simulink model "full car model"  (R2026a)
settings: Solver=VariableStepAuto  StopTime=10
settings Model: Creator=ANDALIBM  LastModifiedBy=eonra
settings SimscapeCC: SimscapeNominalValues="[{\"value\":\"1\",\"unit\":\"A\"},{\"value\":\"1\",\"unit\":\"bar\"},{\"value\":\"1\",\"unit\":\"cm^2\"},{\"value\":\"1\",\"unit\":\"cm^3/s\"},{\"value\":\"1\",\"unit\":\"kJ/kg\"},{\"value\":\"1\",\"unit\":\"kW\"},{\"value\":\"1\",\"unit\":\"l\"},{\"value\":\"1\",\"unit\":\"N\"},{\"value\":\"1\",\"unit\":\"N*m\"},{\"value\":\"1\",\"unit\":\"V\"}]"  SimscapeLogType=none  SimscapeLogDecimation=1  SimscapeLogDataHistory=5000

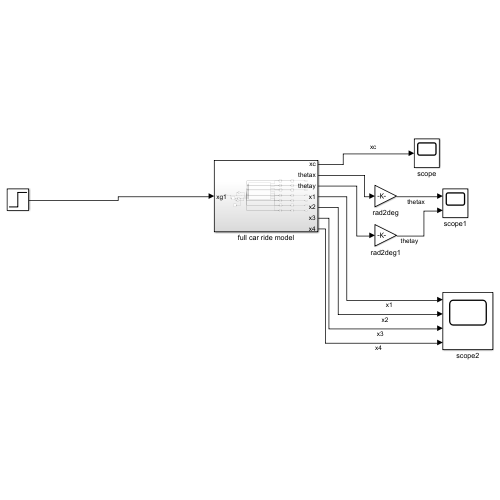
[thumbnail: Simulink's stored preview of the top-level diagram]
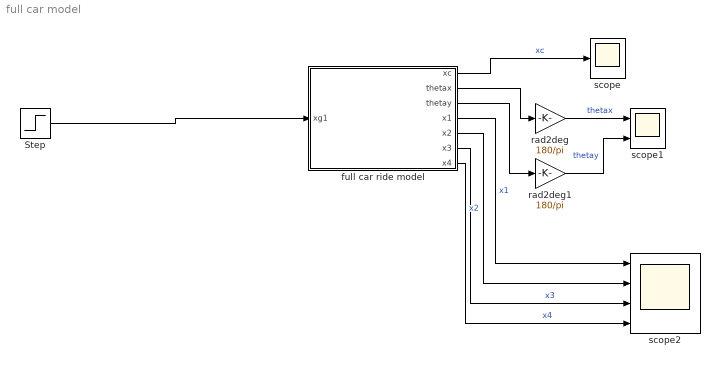
== system full car model ==
  Step : Step  FinalValue=0.05  SampleTime=0
  full car ride model : Subsystem
  rad2deg : Gain  Gain=180/pi
  rad2deg1 : Gain  Gain=180/pi
  scope : Scope
      settings: SampleTime=0.01  ActiveDisplayYMinimum=-0.0065929622757647608  ActiveDisplayYMaximum=0.01986979326753685  DataLoggingVariableName=xc  DataLoggingSaveFormat=Array
  scope1 : Scope  NumInputPorts=2
      settings: SampleTime=0.01  ActiveDisplayYMinimum=-2.6712831731592193  ActiveDisplayYMaximum=0.29680924146213544  DataLoggingSaveFormat=Structure
  scope2 : Scope  NumInputPorts=4
      settings: SampleTime=0.01  ActiveDisplayYMinimum=-0.025734237976273319  ActiveDisplayYMaximum=0.08318787384082596  DataLoggingVariableName=ScopeData2  DataLoggingSaveFormat=Structure
  wires:
  full car ride model/1(xc) -> scope/1  "xc"
  full car ride model/2(thetax) -> rad2deg/1
  rad2deg/1 -> scope1/1  "thetax"
  full car ride model/3(thetay) -> rad2deg1/1
  rad2deg1/1 -> scope1/2  "thetay"
  full car ride model/4(x1) -> scope2/1  "x1"
  full car ride model/7(x4) -> scope2/4  "x4"
  full car ride model/6(x3) -> scope2/3  "x3"
  full car ride model/5(x2) -> scope2/2  "x2"
  Step/1 -> full car ride model/1(xg1)

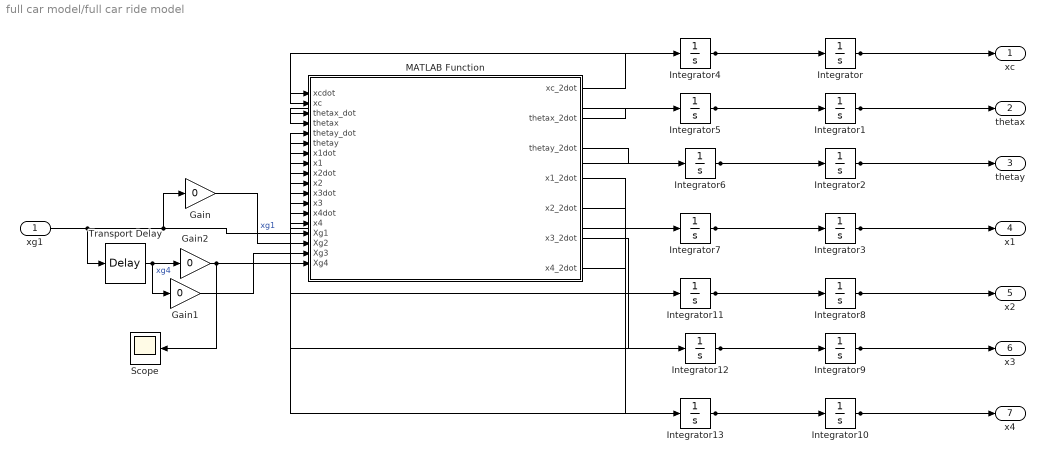
== system full car model/full car ride model ==
  xg1 : Inport
  Gain : Gain  Gain=0
  Gain1 : Gain  Gain=0
  Gain2 : Gain  Gain=0
  Integrator{,1..13} (14 alike) : Integrator
  MATLAB Function : MATLAB Function  TreatAsAtomicUnit=on
  Scope : Scope
      settings: ActiveDisplayYMinimum=-0.0089  ActiveDisplayYMaximum=0.28771  DataLoggingVariableName=ScopeData3
  Transport Delay : TransportDelay  DelayTime=3.1/5
  xc : Outport
  thetax : Outport  Port=2
  thetay : Outport  Port=3
  x1 : Outport  Port=4
  x2 : Outport  Port=5
  x3 : Outport  Port=6
  x4 : Outport  Port=7
  wires:
  Integrator/1 -> xc/1, MATLAB Function/2(xc)
  Integrator1/1 -> thetax/1, MATLAB Function/4(thetax)
  Integrator2/1 -> thetay/1, MATLAB Function/6(thetay)
  Integrator3/1 -> x1/1, MATLAB Function/8(x1)
  Integrator7/1 -> Integrator3/1, MATLAB Function/7(x1dot)
  Integrator6/1 -> Integrator2/1, MATLAB Function/5(thetay_dot)
  Integrator5/1 -> Integrator1/1, MATLAB Function/3(thetax_dot)
  Integrator4/1 -> Integrator/1, MATLAB Function/1(xcdot)
  xg1/1 -> Gain/1, MATLAB Function/15(Xg1), Transport Delay/1  "xg1"
  Transport Delay/1 -> Gain1/1, Gain2/1  "xg4"
  Integrator11/1 -> Integrator8/1, MATLAB Function/9(x2dot)
  Integrator12/1 -> Integrator9/1, MATLAB Function/11(x3dot)
  Integrator13/1 -> Integrator10/1, MATLAB Function/13(x4dot)
  Integrator10/1 -> x4/1, MATLAB Function/14(x4)
  Integrator9/1 -> x3/1, MATLAB Function/12(x3)
  Integrator8/1 -> x2/1, MATLAB Function/10(x2)
  MATLAB Function/1(xc_2dot) -> Integrator4/1
  MATLAB Function/2(thetax_2dot) -> Integrator5/1
  MATLAB Function/3(thetay_2dot) -> Integrator6/1
  MATLAB Function/4(x1_2dot) -> Integrator7/1
  MATLAB Function/5(x2_2dot) -> Integrator11/1
  MATLAB Function/6(x3_2dot) -> Integrator12/1
  MATLAB Function/7(x4_2dot) -> Integrator13/1
  Gain/1 -> MATLAB Function/16(Xg2)
  Gain1/1 -> MATLAB Function/17(Xg3)
  Gain2/1 -> MATLAB Function/18(Xg4), Scope/1

== matlab function full car model/full car ride model/MATLAB Function ==
  data: xcdot input; xc input; thetax_dot input; thetax input; thetay_dot input; thetay input; x1dot input; xc_2dot output; x1 input; thetax_2dot output; thetay_2dot output; x1_2dot output; x2_2dot output; x2dot input; x2 input; x3dot input; x3 input; x4dot input; x4 input; Xg1 input; Xg2 input; Xg3 input; Xg4 input; x3_2dot output; x4_2dot output
function [xc_2dot,thetax_2dot,thetay_2dot,x1_2dot,x2_2dot,x3_2dot,x4_2dot] = fcn(xcdot,xc,thetax_dot,thetax,...
    thetay_dot,thetay,x1dot,x1,x2dot,x2,x3dot,x3,x4dot,x4,Xg1,Xg2,Xg3,Xg4)

a=0.8;
b=0.8;
c=0.6;
d=0.6;
M=300;
Ixx=90;
Iyy=120;
m1=20;
m2=20;
m3=20;
m4=20;
K1=15000;
K2=15000;
K3=15000;
K4=15000;
C1=3000;
C2=3000;
C3=3000;
C4=3000;
Kt1=200000;
Kt2=200000;
Kt3=200000;
Kt4=200000;

xc_2dot=(K1*(x1-(-a*thetay-c*thetax+xc))+C1*(x1dot-(-a*thetay_dot-c*thetax_dot+xcdot))+...
         K2*(x2-(-a*thetay+d*thetax+xc))+C2*(x2dot-(-a*thetay_dot+d*thetax_dot+xcdot))+...
         K3*(x3-(b*thetay+d*thetax+xc))+C3*(x3dot-(b*thetay_dot+d*thetax_dot+xcdot))+...
         K4*(x4-(b*thetay-c*thetax+xc))+C4*(x4dot-(b*thetay_dot-c*thetax_dot+xcdot)))/M;

thetax_2dot=(d*(K2*(x2-(-a*thetay+d*thetax+xc))+C2*(x2dot-(-a*thetay_dot+d*thetax_dot+xcdot))+...
         K3*(x3-(b*thetay+d*thetax+xc))+C3*(x3dot-(b*thetay_dot+d*thetax_dot+xcdot)))-...
         c*(K1*(x1-(-a*thetay-c*thetax+xc))+C1*(x1dot-(-a*thetay_dot-c*thetax_dot+xcdot))+...
         K4*(x4-(b*thetay-c*thetax+xc))+C4*(x4dot-(b*thetay_dot-c*thetax_dot+xcdot))))/Ixx;

thetay_2dot=(b*(K4*(x4-(b*thetay-c*thetax+xc))+C4*(x4dot-(b*thetay_dot-c*thetax_dot+xcdot))+...
         K3*(x3-(b*thetay+d*thetax+xc))+C3*(x3dot-(b*thetay_dot+d*thetax_dot+xcdot)))-...
         a*(K1*(x1-(-a*thetay-c*thetax+xc))+C1*(x1dot-(-a*thetay_dot-c*thetax_dot+xcdot))+...
         K1*(x1-(-a*thetay-c*thetax+xc))+C1*(x1dot-(-a*thetay_dot-c*thetax_dot+xcdot))))/Ixx;

x1_2dot=(-K1*(x1-(-a*thetay-c*thetax+xc))-C1*(x1dot-(-a*thetay_dot-c*thetax_dot+xcdot))+Kt1*(Xg1-x1))/m1;

x2_2dot=(-K2*(x2-(-a*thetay+d*thetax+xc))-C2*(x2dot-(-a*thetay_dot+d*thetax_dot+xcdot))+Kt2*(Xg2-x2))/m2;

x3_2dot=(-K3*(x3-(b*thetay+d*thetax+xc))-C3*(x3dot-(b*thetay_dot+d*thetax_dot+xcdot))+Kt3*(Xg3-x3))/m3;

x4_2dot=(-K4*(x4-(b*thetay-c*thetax+xc))-C4*(x4dot-(b*thetay_dot-c*thetax_dot+xcdot))+Kt4*(Xg4-x4))/m4;
